simulink model "MagLev_Controller_Design"  (R2020b)
settings: Solver=ode5  StartTime=0.0  StopTime=2  FixedStep=0.0001  RelTol=1e-3
undefined symbols (not defined in the file or in its folder): actuator_gain, K, p, sensor_gain, v_bias, v_ref, z
settings Model: Creator=aanan  LastModifiedBy=aanan
settings DataIOCC: SaveFormat=Array  SignalLogging=off  DSMLogging=off  ReturnWorkspaceOutputs=off

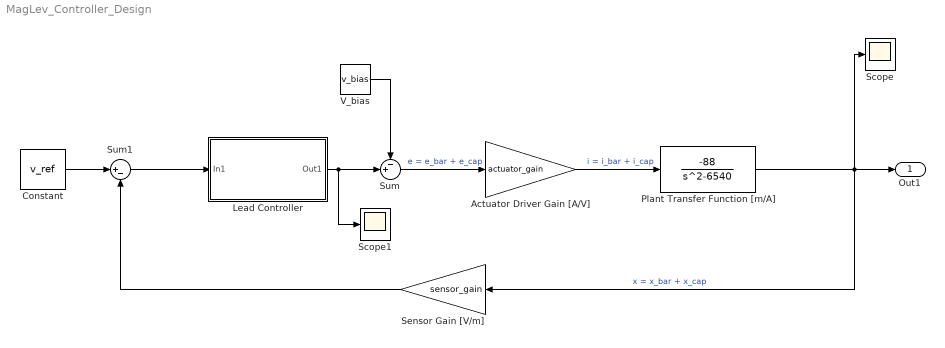
== system MagLev_Controller_Design ==
  Actuator Driver Gain [A/V] : Gain  Gain=actuator_gain
  Constant : Constant  Value=v_ref
  Lead Controller : Subsystem
  Plant Transfer Function [m/A] : TransferFcn  Numerator=[-88]  Denominator=[1 0 -6540]
  Scope : Scope
  Scope1 : Scope
  Sensor Gain [V/m] : Gain  Gain=sensor_gain
  Sum : Sum  Inputs=-+|
  Sum1 : Sum  Inputs=|+-
  V_bias : Constant  Value=v_bias
  Out1 : Outport
  wires:
  V_bias/1 -> Sum/1
  Sum/1 -> Actuator Driver Gain [A/V]/1  "e = e_bar + e_cap"
  Actuator Driver Gain [A/V]/1 -> Plant Transfer Function [m/A]/1  "i = i_bar + i_cap"
  Plant Transfer Function [m/A]/1 -> Scope/1, Out1/1, Sensor Gain [V/m]/1  "x = x_bar + x_cap"
  Sensor Gain [V/m]/1 -> Sum1/2
  Constant/1 -> Sum1/1
  Sum1/1 -> Lead Controller/1(In1)
  Lead Controller/1(Out1) -> Scope1/1, Sum/2

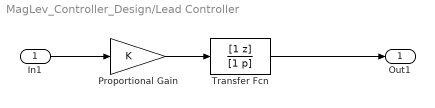
== system MagLev_Controller_Design/Lead Controller ==
  In1 : Inport
  Proportional Gain : Gain  Gain=K
  Transfer Fcn : TransferFcn  Numerator=[1 z]  Denominator=[1 p]
  Out1 : Outport
  wires:
  In1/1 -> Proportional Gain/1
  Transfer Fcn/1 -> Out1/1
  Proportional Gain/1 -> Transfer Fcn/1
